simulink model "MSDcont"  (R2018a)
settings: Solver=ode15s  StartTime=0.0  StopTime=Tsim  MaxStep=0.01  RelTol=1e-3
values from neighbouring files (symbols this model uses):
  A = [    0    1 ... (first row only)    [massSpringDamper_LQR.m]    (also in msd_least_squares.m = [0    1; -k/m  -c/m]; symbolic_msd.m = [0 1; (-omega_n^2) (-2*omega_n*zeta)])
  B = [ 0 ; 1/m]    [massSpringDamper_LQR.m]    (also in msd_least_squares.m; symbolic_msd.m = [0;1/m])
  H = H(1)    [massSpringDamper_LQR.m]    (also in msd_least_squares.m = zeros(101,2))
  x0 = [0;0]    [massSpringDamper_LQR.m]    (also in msd_least_squares.m)
settings Model: Creator=dicairano  LastModifiedBy=srivats
settings CodeAppCC: StateflowObjectComments=on

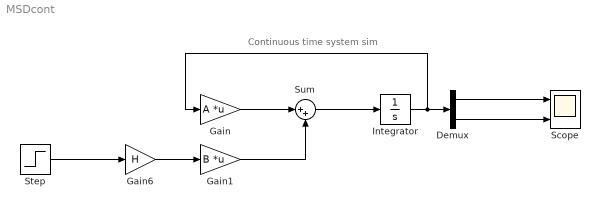
== system MSDcont ==
  note: Continuous time system sim
  Demux : Demux  Outputs=2
  Gain : Gain  Gain=A  Multiplication=Matrix(K*u)
  Gain1 : Gain  Gain=B  Multiplication=Matrix(K*u)
  Gain6 : Gain  Gain=H
  Integrator : Integrator  InitialCondition=x0
  Scope : Scope  NumInputPorts=2
  Step : Step  Time=0  SampleTime=0
  Sum : Sum  Inputs=|++
  wires:
  Gain/1 -> Sum/1
  Sum/1 -> Integrator/1
  Gain1/1 -> Sum/2
  Integrator/1 -> Demux/1, Gain/1
  Demux/1 -> Scope/1
  Demux/2 -> Scope/2
  Gain6/1 -> Gain1/1
  Step/1 -> Gain6/1
